simulink model "OPC_UA_Test"  (R2024b)
settings: Solver=FixedStepDiscrete  StartTime=0.0  StopTime=inf  FixedStep=0.01  MaxStep=0.001  RelTol=1e-3
libraries: opcualib x1, sldrtlib x1
settings Model: Creator=Green Crane Testbed  LastModifiedBy=Green Crane Testbed

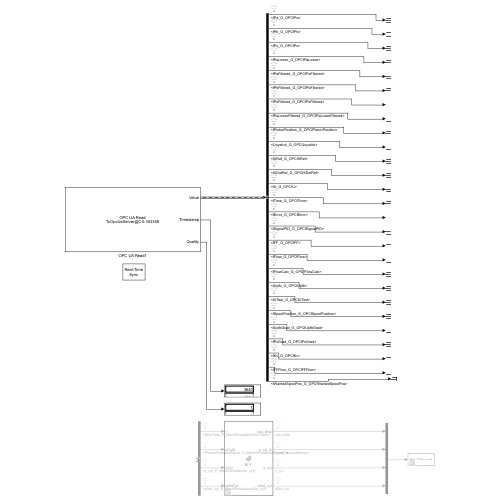
[thumbnail: Simulink's stored preview of the top-level diagram]
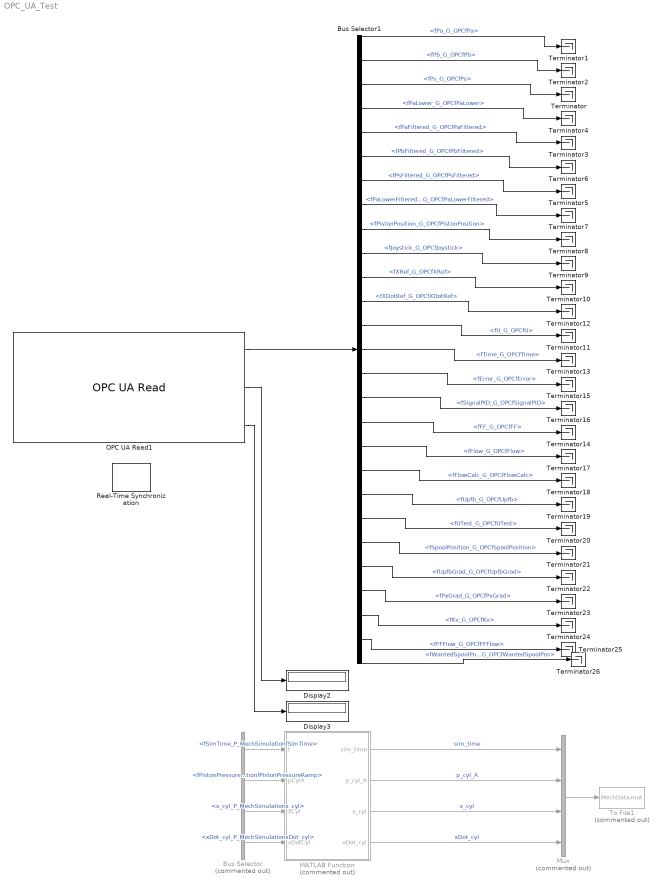
== system OPC_UA_Test ==
  Bus Selector : BusSelector  Commented=on  OutputSignals=fSimTime_P_MechSimulationfSimTime,fPistonPressureRamp_P_MechSimulationfPistonPressureRamp,x_cyl_P_MechSimulationx_cyl,xDot_cyl_P_MechSimulationxDot_cyl
  Bus Selector1 : BusSelector  OutputSignals=fPa_G_OPCfPa,fPb_G_OPCfPb,fPs_G_OPCfPs,fPaLower_G_OPCfPaLower,fPaFiltered_G_OPCfPaFiltered,fPbFiltered_G_OPCfPbFiltered,fPsFiltered_G_OPCfPsFiltered,fPaLowerFiltered_G_OPCfPaLowerFiltered,fPistonPosition_G_OPCfPistonPosition,fJoystick_G_OPCfJoystick,fXRef_G_OPCfXRef,fXDotRef_G_OPCfXDotRef,fU_G_OPCfU,fTime_G_OPCfTime,fError_G_OPCfError,fSignalPID_G_OPCfSignalPID,fFF_G_OPCfFF,fFlow_G_OPCfFlow,fFlowCalc_G_OPCfFlowCalc,fUpfb_G_OPCfUpfb,fUTest_G_OPCfUTest,fSpoolPosition_G_OPCfSpoolPosition,fUpfbGrad_G_OPCfUpfbGrad,fPxGrad_G_OPCfPxGrad,fKv_G_OPCfKv,fFFFlow_G_OPCfFFFlow,fWantedSpoolPos_G_OPCfWantedSpoolPos
  Display2 : Display
  Display3 : Display
  MATLAB Function : MATLAB Function  Commented=on  TreatAsAtomicUnit=on
  Mux : Mux  Commented=on
  OPC UA Read1 : opcualib/OPC UA Read  SelectedServer=TcOpcUaServer@CX-353358  ServerList=TcOpcUaServer@CX-353358  NodeList={ '1', 'fPa', '4', 'G_OPC.fPa', '0'; '2', 'fPb', '4', 'G_OPC.fPb', '0'; '3', 'fPs', '4', 'G_OPC.fPs', '0'; '4', 'fPaLower', '4', 'G_OPC.fPaLower', '0'; '5', 'fPaFiltered', '4', 'G_OPC.fPaFiltered', '0'; '6', 'fPbFiltered', '4', 'G_OPC.fPbFiltered', '0'; '7', 'fPsFiltered', '4', 'G_OPC.fPsFiltered', '0'; '8', 'fPaLowerFiltered', '4', 'G_OPC.fPaLowerFiltered', '0'; '9', 'fSpoolPosition', '4', 'G_OPC.fSpoolPosition', '0'; '10', 'fPistonPosition', '4', 'G_OPC.fPistonPosition', '0'; '11', 'fJoystick', '4', 'G_OPC.fJoystick', '0'; '12', 'fFlow', '4', 'G_OPC.fFlow', '0'; '13', 'fFlowCalc', '4', 'G_OPC.fFlowCalc', '0'; '14', 'fXRef', '4', 'G_OPC.fXRef', '0'; '15', 'fXDotRef', '4', 'G_OPC.fXDotRef', '0'; '16', 'fU', '4', 'G_OPC.fU', '0'; '17', 'fUpfb', '4', 'G_OPC.fUpfb', '0'; '18', 'fUTest', '4', 'G_OPC.fUTest', '0'; '19', 'fTime', '4', 'G_OPC.fTime', '0'; '20', 'fError', '4', 'G_OPC.fError', '0'; '21', 'fSignalPID', '4', 'G_OPC.fSignalPID', '0'; '22', 'fFF', '4', 'G_OPC.fFF', '0'; '23', 'fUpfbGrad', '4', 'G_OPC.fUpfbGrad', '0'; '24', 'fPxGrad', '4', 'G_OPC.fPxGrad', '0'; '25', 'fKv', '4', 'G_OPC.fKv', '0'; '26', 'fFFFlow', '4', 'G_OPC.fFFFlow', '0'; '27', 'fWantedSpoolPos', '4', 'G_OPC.fWantedSpoolPos', '0' }  ShowQualityPort=on  ShowTimestampPort=on  ShowTimestampPortAs=Seconds since start  SampleTime=-1
  Real-Time Synchronization : sldrtlib/Real-Time Synchronization  SampleTime=-1  MaxMissedTicks=1000000000000  ShowMissedTicks=off  YieldWhenWaiting=off
  Terminator{,1..26} (27 alike) : Terminator
  To File1 : ToFile  Commented=on  Filename=MechData.mat  SaveFormat=Timeseries
  wires:
  Mux/1 -> To File1/1
  Bus Selector1/23 -> Terminator22/1  "<fUpfbGrad_G_OPCfUpfbGrad>"
  OPC UA Read1/1 -> Bus Selector1/1
  OPC UA Read1/3 -> Display3/1
  OPC UA Read1/2 -> Display2/1
  Bus Selector/2 -> MATLAB Function/2(pCylA)  "<fPistonPressureRamp_P_MechSimulationfPistonPressureRamp>"
  Bus Selector/4 -> MATLAB Function/4(xDotCyl)  "<xDot_cyl_P_MechSimulationxDot_cyl>"
  Bus Selector/1 -> MATLAB Function/1(t)  "<fSimTime_P_MechSimulationfSimTime>"
  Bus Selector/3 -> MATLAB Function/3(xCyl)  "<x_cyl_P_MechSimulationx_cyl>"
  Bus Selector1/5 -> Terminator3/1  "<fPaFiltered_G_OPCfPaFiltered>"
  Bus Selector1/3 -> Terminator/1  "<fPs_G_OPCfPs>"
  Bus Selector1/1 -> Terminator1/1  "<fPa_G_OPCfPa>"
  Bus Selector1/6 -> Terminator6/1  "<fPbFiltered_G_OPCfPbFiltered>"
  Bus Selector1/4 -> Terminator4/1  "<fPaLower_G_OPCfPaLower>"
  Bus Selector1/2 -> Terminator2/1  "<fPb_G_OPCfPb>"
  Bus Selector1/13 -> Terminator11/1  "<fU_G_OPCfU>"
  Bus Selector1/11 -> Terminator10/1  "<fXRef_G_OPCfXRef>"
  Bus Selector1/9 -> Terminator8/1  "<fPistonPosition_G_OPCfPistonPosition>"
  Bus Selector1/7 -> Terminator5/1  "<fPsFiltered_G_OPCfPsFiltered>"
  Bus Selector1/14 -> Terminator13/1  "<fTime_G_OPCfTime>"
  Bus Selector1/12 -> Terminator12/1  "<fXDotRef_G_OPCfXDotRef>"
  Bus Selector1/10 -> Terminator9/1  "<fJoystick_G_OPCfJoystick>"
  Bus Selector1/8 -> Terminator7/1  "<fPaLowerFiltered_G_OPCfPaLowerFiltered>"
  Bus Selector1/25 -> Terminator24/1  "<fKv_G_OPCfKv>"
  Bus Selector1/15 -> Terminator15/1  "<fError_G_OPCfError>"
  Bus Selector1/16 -> Terminator16/1  "<fSignalPID_G_OPCfSignalPID>"
  Bus Selector1/21 -> Terminator20/1  "<fUTest_G_OPCfUTest>"
  Bus Selector1/19 -> Terminator18/1  "<fFlowCalc_G_OPCfFlowCalc>"
  Bus Selector1/17 -> Terminator14/1  "<fFF_G_OPCfFF>"
  Bus Selector1/26 -> Terminator25/1  "<fFFFlow_G_OPCfFFFlow>"
  Bus Selector1/20 -> Terminator19/1  "<fUpfb_G_OPCfUpfb>"
  Bus Selector1/18 -> Terminator17/1  "<fFlow_G_OPCfFlow>"
  Bus Selector1/22 -> Terminator21/1  "<fSpoolPosition_G_OPCfSpoolPosition>"
  Bus Selector1/24 -> Terminator23/1  "<fPxGrad_G_OPCfPxGrad>"
  MATLAB Function/3(x_cyl) -> Mux/3  "x_cyl"
  MATLAB Function/1(sim_time) -> Mux/1  "sim_time"
  MATLAB Function/4(xDot_cyl) -> Mux/4  "xDot_cyl"
  MATLAB Function/2(p_cyl_A) -> Mux/2  "p_cyl_A"
  Bus Selector1/27 -> Terminator26/1  "<fWantedSpoolPos_G_OPCfWantedSpoolPos>"

== matlab function OPC_UA_Test/MATLAB Function ==
  data: t input; sim_time output; p_cyl_A output; x_cyl output; xDot_cyl output; pCylA input; xCyl input; xDotCyl input
function [sim_time, p_cyl_A, x_cyl, xDot_cyl]   = fcn(t, pCylA, xCyl, xDotCyl)
if t >= 0.0 && t < 10.0
     sim_time = t;
     p_cyl_A = pCylA;
     x_cyl = xCyl;
     xDot_cyl = xDotCyl;
elseif t >= 10.0
     sim_time = 10.0;
     p_cyl_A = pCylA;
     x_cyl = xCyl;
     xDot_cyl = xDotCyl;
else
     sim_time = 0.0;
     p_cyl_A = 0.0;
     x_cyl = 0.0;
     xDot_cyl = 0.0;
end
